simulink model "three_phase_full_wave_ac_voltage_controller"  (R2024a)
settings: Solver=ode23tb  StartTime=0.0  StopTime=0.04  MaxStep=1e-4  RelTol=1e-3
libraries: spsThyristorLib x6, spsVoltageMeasurementLib x3, spsRMSLib x3, spsSeriesRLCBranchLib x3, spsGroundLib x1, spsThreePhaseSourceLib x1, sps_lib x1
settings Model: Creator=Shiyam  LastModifiedBy=Asus
settings SolverCC: AlgebraicLoopSolver=TrustRegion
settings DebuggingCC: UnconnectedInputMsg=warning  UnconnectedOutputMsg=warning  UnconnectedLineMsg=warning
settings ModelReferenceCC: EnableRefExpFcnMdlSchedulingChecks=on
settings SFSimCC: CustomCodeUndefinedFunction=UseInterfaceOnly
settings RTWCC: GPUComputeCapability=3.5

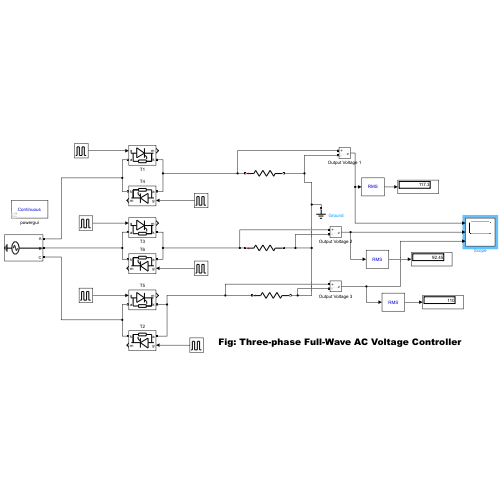
[thumbnail: Simulink's stored preview of the top-level diagram]
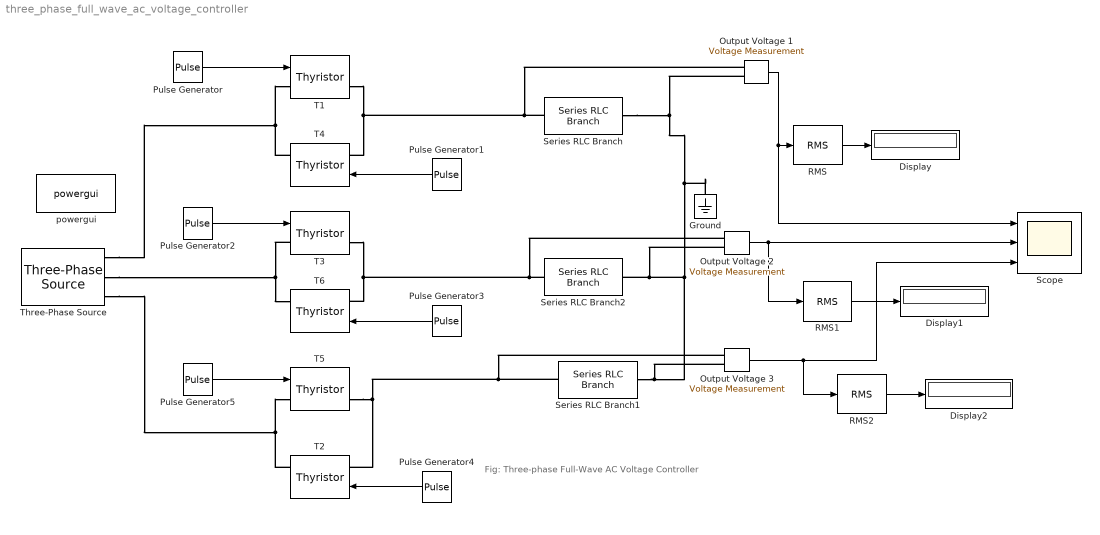
== system three_phase_full_wave_ac_voltage_controller ==
  note: Fig: Three-phase Full-Wave AC Voltage Controller
  Display : Display
  Display1 : Display
  Display2 : Display
  Ground : spsGroundLib/Ground  LConnTagsString=a
  Output Voltage 1 : spsVoltageMeasurementLib/Voltage Measurement  PhasorSimulation=off  OutputType=Complex  PSBequivalent=0
  Output Voltage 2 : spsVoltageMeasurementLib/Voltage Measurement  PhasorSimulation=off  OutputType=Complex  PSBequivalent=0
  Output Voltage 3 : spsVoltageMeasurementLib/Voltage Measurement  PhasorSimulation=off  OutputType=Complex  PSBequivalent=0
  Pulse Generator : DiscretePulseGenerator  PulseType=Time based  Period=0.02  PulseWidth=60  PhaseDelay=60*(.02/360)
  Pulse Generator1 : DiscretePulseGenerator  PulseType=Time based  Period=0.02  PulseWidth=60  PhaseDelay=(60+180)*(.02/360)
  Pulse Generator2 : DiscretePulseGenerator  PulseType=Time based  Period=0.02  PulseWidth=60  PhaseDelay=(60+120)*(.02/360)
  Pulse Generator3 : DiscretePulseGenerator  PulseType=Time based  Period=0.02  PulseWidth=60  PhaseDelay=(60+300)*(.02/360)
  Pulse Generator4 : DiscretePulseGenerator  PulseType=Time based  Period=0.02  PulseWidth=60  PhaseDelay=(60+60)*(.02/360)
  Pulse Generator5 : DiscretePulseGenerator  PulseType=Time based  Period=0.02  PulseWidth=60  PhaseDelay=(60+240)*(.02/360)
  RMS : spsRMSLib/RMS  TrueRMS=on  Freq=60  RMSInit=120  Ts=0
  RMS1 : spsRMSLib/RMS  TrueRMS=on  Freq=60  RMSInit=120  Ts=0
  RMS2 : spsRMSLib/RMS  TrueRMS=on  Freq=60  RMSInit=120  Ts=0
  Scope : Scope  NumInputPorts=3
  Series RLC Branch : spsSeriesRLCBranchLib/Series RLC Branch  LConnTagsString=__new0  RConnTagsString=__new0  BranchType=R  Resistance=10  Inductance=1e-3  SetiL0=off  InitialCurrent=0  Capacitance=1e-6  Setx0=off  InitialVoltage=0  Measurements=None
  Series RLC Branch1 : spsSeriesRLCBranchLib/Series RLC Branch  LConnTagsString=__new0  RConnTagsString=__new0  BranchType=R  Resistance=10  Inductance=1e-3  SetiL0=off  InitialCurrent=0  Capacitance=1e-6  Setx0=off  InitialVoltage=0  Measurements=None
  Series RLC Branch2 : spsSeriesRLCBranchLib/Series RLC Branch  LConnTagsString=__new0  RConnTagsString=__new0  BranchType=R  Resistance=10  Inductance=1e-3  SetiL0=off  InitialCurrent=0  Capacitance=1e-6  Setx0=off  InitialVoltage=0  Measurements=None
  T{1..6} (6 alike) : spsThyristorLib/Thyristor  Ron=0.001  Lon=0  Vf=0.8  IC=0  Rs=500  Cs=250e-9  Measurements=on
  Three-Phase Source : spsThreePhaseSourceLib/Three-Phase Source  InternalConnection=Yg  VoltagePhases=on  Voltage=25e3  PhaseAngle=0  Voltage_phases=[208 208 208]/sqrt(3)  PhaseAngles_phases=[0 -120 +120]  Frequency=50  NonIdealSource=off  SpecifyImpedance=off  Resistance=0.8929  Inductance=16.58e-3  ShortCircuitLevel=100e6  BaseVoltage=25e3  XRratio=7  BusType=swing  Pref=10e3  Qref=0  Prefabc=[10e3, 10e3, 10e3]  Qrefabc=[0, 0, 0]  Qmin=-inf  Qmax=inf
  powergui : sps_lib/powergui  Priority=1  SimulationMode=Continuous  SampleTime=50e-6  frequency=60  Iterations=50  frequencyindice=50  Pbase=100e6  ErrMax=1e-4  UnitsV=kV  UnitsW=MW  buscounter=0  FunctionMessages=off  echomessages=off  EnableUseOfTLC=off  CurrentSourceSwitches=off  DisableSnubberDevices=off  DisableRonSwitches=off  DisableVfSwitches=off  DisplayEquations=off  AutomaticDiscreteSolvers=off  SolverType=Tustin/Backward Euler (TBE)  Interpol=off  ExternalGateDelay=off  methode=off  Ts=100  x0status=blocks  SPID=on  SwTol=0  HookPort=off  NonlinearTolerance=0  nMaxIteration=15  ContinueOnMaxIteration=off  RestoreLinks=warning  ResistiveCurrentMeasurement=off  Frange=[0:2:500]  Ylog=off  Xlog=on  ShowGrid=off  save=off  variable=ZData  structure=0  ZoomFFT=off  StartTime=0.0  cycles=1  DisplayStyle=1  fundamental=60  FreqAxis=off  MaxFrequency=1000  frequencyindicesteady=1  RmsSteady=1  display=off
  wires:
  Pulse Generator3/1 -> T6/1
  Pulse Generator5/1 -> T5/1
  Output Voltage 1/1 -> Scope/1, RMS/1
  Pulse Generator2/1 -> T3/1
  Pulse Generator/1 -> T1/1
  Pulse Generator1/1 -> T4/1
  Pulse Generator4/1 -> T2/1
  RMS/1 -> Display/1
  Output Voltage 2/1 -> RMS1/1, Scope/2
  RMS1/1 -> Display1/1
  Output Voltage 3/1 -> Scope/3, RMS2/1
  RMS2/1 -> Display2/1
  connections:
  Series RLC Branch/RConn1 -- Ground/LConn1 -- Output Voltage 3/LConn2 -- Series RLC Branch1/RConn1 -- Output Voltage 2/LConn2 -- Series RLC Branch2/RConn1 -- Output Voltage 1/LConn2
  T5/RConn1 -- Output Voltage 3/LConn1 -- Series RLC Branch1/LConn1 -- T2/LConn1
  T4/LConn1 -- T1/RConn1 -- Output Voltage 1/LConn1 -- Series RLC Branch/LConn1
  T2/RConn1 -- Three-Phase Source/RConn3 -- T5/LConn1
  T4/RConn1 -- Three-Phase Source/RConn1 -- T1/LConn1
  T6/LConn1 -- Output Voltage 2/LConn1 -- Series RLC Branch2/LConn1 -- T3/RConn1
  T3/LConn1 -- Three-Phase Source/RConn2 -- T6/RConn1
